simulink model "SystemBlockDiagram"  (R2024b)
settings: Solver=VariableStepAuto  StartTime=0.0  StopTime=10.0  RelTol=1e-3
settings Model: Creator=Fady  LastModifiedBy=Fady

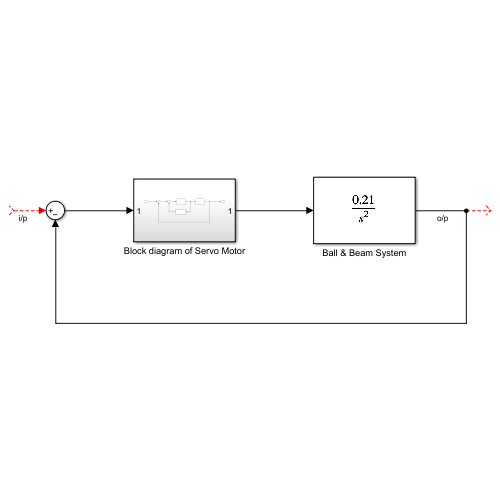
[thumbnail: Simulink's stored preview of the top-level diagram]
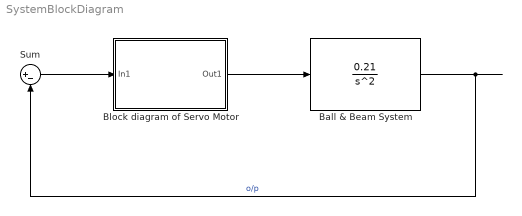
== system SystemBlockDiagram ==
  Ball & Beam System : TransferFcn  Numerator=[0.21]  Denominator=[1 0 0]
  Block diagram of Servo Motor : Subsystem
  Sum : Sum  Inputs=|+-
  wires:
  Block diagram of Servo Motor/1(Out1) -> Ball & Beam System/1
  Sum/1 -> Block diagram of Servo Motor/1(In1)
  Ball & Beam System/1 -> Sum/2  "o/p"
  ? -> Sum/1  "i/p"

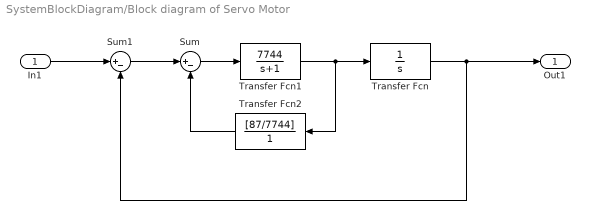
== system SystemBlockDiagram/Block diagram of Servo Motor ==
  In1 : Inport
  Sum : Sum  Inputs=|+-
  Sum1 : Sum  Inputs=|+-
  Transfer Fcn : TransferFcn  Denominator=[1 0]
  Transfer Fcn1 : TransferFcn  Numerator=[7744]  Denominator=[1 1]
  Transfer Fcn2 : TransferFcn  Numerator=[87/7744]  Denominator=[1]
  Out1 : Outport
  wires:
  Transfer Fcn/1 -> Out1/1, Sum1/2
  Transfer Fcn1/1 -> Transfer Fcn2/1, Transfer Fcn/1
  Sum1/1 -> Sum/1
  Sum/1 -> Transfer Fcn1/1
  Transfer Fcn2/1 -> Sum/2
  In1/1 -> Sum1/1
